simulink library "PMV_PPD"  (R2018b)
settings: Solver=ode45  StartTime=0.0  StopTime=10.0  RelTol=1e-3  EnableMultiTasking=on
undefined symbols (not defined in the file): CarnotCallbacks_PMV_PPD
settings Model: Creator=drhf  LastModifiedBy=drhf
settings DataIOCC: LimitDataPoints=on  SaveFormat=Array  SignalLoggingSaveFormat=ModelDataLogs
settings OptimizationCC: ExpressionDepthLimit=2147483647  LifeSpan=inf
settings DebuggingCC: UnderspecifiedInitializationDetection=Classic  MergeDetectMultiDrivingBlocksExec=none  SolverPrmCheckMsg=warning  FcnCallInpInsideContextMsg=warning  StateNameClashWarn=warning  SFUnexpectedBacktrackingDiag=warning  SFNoUnconditionalDefaultTransitionDiag=warning  SFExecutionAtInitializationDiag=none
settings HardwareCC: ProdBitPerPointer=32  ProdBitPerSizeT=32  ProdBitPerPtrDiffT=32  ProdLargestAtomicFloat=None  ProdIntDivRoundTo=Undefined  ProdEndianess=Unspecified  ProdWordSize=32  ProdHWDeviceType=32-bit Generic
settings ModelReferenceCC: PropagateSignalLabelsOutOfModel=off
settings SFSimCC: SimUseLocalCustomCode=off
settings RTWCC: RTWUseLocalCustomCode=off
settings CodeAppCC: StateflowObjectComments=on
settings GRTTargetCC: TargetLangStandard=C89/C90 (ANSI)  GeneratePreprocessorConditionals=Disable all  CombineOutputUpdateFcns=off  GRTInterface=on
settings ConfigComp: CovMetricSettings=dw  CovHtmlReporting=on  CovSaveCumulativeToWorkspaceVar=on  CovSaveSingleToWorkspaceVar=on  CovExternalEMLEnable=off

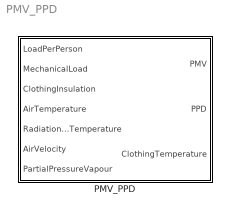
== system PMV_PPD ==
  PMV_PPD : Subsystem  LoadFcn=CarnotCallbacks_PMV_PPD('LoadFcn', gcb);  mask(PMV_PPD){DEBUGLEVEL=WARNINGLEVEL, MAXTOTALWARNINGS=inf, MAXCONSECUTIVEWARNINGS=inf, WRITETOFILE=0, FILENAME='messages.txt'}
      mask prompts: DEBUGLEVEL "Debug level"; MAXTOTALWARNINGS "maximum number of total warning"; MAXCONSECUTIVEWARNINGS "maximum number of consecutive warnings"; WRITETOFILE "write messages to file"; FILENAME "filename for messages"
      mask help:
      | This block calculates from it's inputs the thermal comfort according to PMV (pedicted mean vote) and PPD (predicted percentage of dissatisfied).
      | LoadPerPerson : metabolic rate of persons per surface in W/m² (typical 58.2 W/m²)
      | MechanicalLoad : effective mechanical power of a person in W/m²
      | ClothingIsolation : thermal resistance of the clothing in [m²/kW]; 1 clo = 0.155 W/m²
      | air temperature [°C]
      | radiation temperature [°C]
      | relative air velocity [m/s]
      | PartialPressureVapur : partial pressure of water [Pa]
      mask init:
      | %global debug level
      | [DEBUGLEVEL, MAXTOTALWARNINGS, MAXCONSECUTIVEWARNINGS, WRITETOFILE, FILENAME] = CarnotCallbacks_PMV_PPD('CheckDebugLevels', DEBUGLEVEL, MAXTOTALWARNINGS, MAXCONSECUTIVEWARNINGS, WRITETOFILE, FILENAME);
      mask Help: web(fullfile(path_carnot('help'),'PMV_PPD.html'),'-helpbrowser')
      mask TypeOptions DEBUGLEVEL: DEBUGLEVEL | INFOLEVEL | WARNINGLEVEL | ERRORLEVEL | FATALLEVEL | NOLEVEL
      mask Callback DEBUGLEVEL: CarnotCallbacks_PMV_PPD('MaskVisibilities');
      mask DialogControl ParameterTabVar0 Prompt: debugging air property calculations

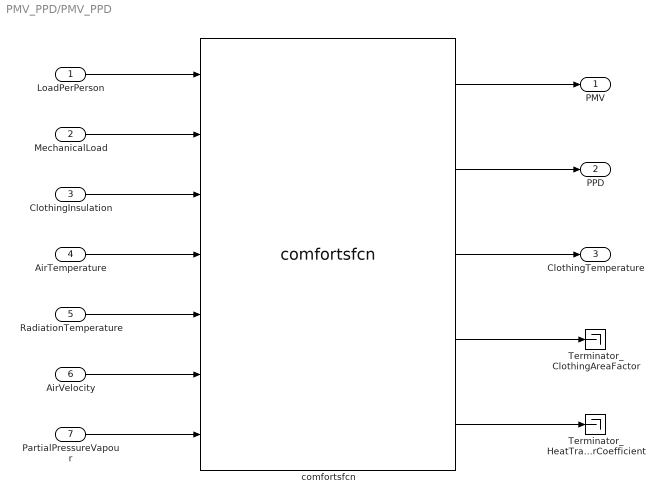
== system PMV_PPD/PMV_PPD ==
  LoadPerPerson : Inport
  MechanicalLoad : Inport  Port=2
  ClothingInsulation : Inport  Port=3
  AirTemperature : Inport  Port=4
  RadiationTemperature : Inport  Port=5
  AirVelocity : Inport  Port=6
  PartialPressureVapour : Inport  Port=7
  Terminator_ClothingAreaFactor : Terminator
  Terminator_HeatTransferCoefficient : Terminator
  comfortsfcn : S-Function  FunctionName=comfortsfcn  Parameters=DEBUGLEVEL-1, MAXTOTALWARNINGS, MAXCONSECUTIVEWARNINGS, WRITETOFILE, FILENAME  SFunctionDeploymentMode=off  EnableBusSupport=off
  PMV : Outport
  PPD : Outport  Port=2
  ClothingTemperature : Outport  Port=3
  wires:
  PartialPressureVapour/1 -> comfortsfcn/7
  AirTemperature/1 -> comfortsfcn/4
  LoadPerPerson/1 -> comfortsfcn/1
  MechanicalLoad/1 -> comfortsfcn/2
  ClothingInsulation/1 -> comfortsfcn/3
  RadiationTemperature/1 -> comfortsfcn/5
  AirVelocity/1 -> comfortsfcn/6
  comfortsfcn/1 -> PMV/1
  comfortsfcn/2 -> PPD/1
  comfortsfcn/3 -> ClothingTemperature/1
  comfortsfcn/4 -> Terminator_ClothingAreaFactor/1
  comfortsfcn/5 -> Terminator_HeatTransferCoefficient/1
